simulink model "sim_test2"  (R2018a)
settings: Solver=FixedStepDiscrete  StartTime=0.0  StopTime=2e-3  FixedStep=Ts  RelTol=1e-3
InitFcn:
  | clear all;
  | close all;
  | clc;
  | 
  | Ts = 0.01e-3;  % sample period = 0.1 ms
  | Fs = 1/Ts;     % sample rate = 10kHz
settings Model: Creator=Ryan  LastModifiedBy=Ryan

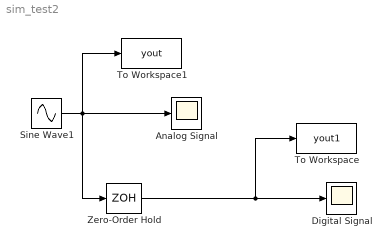
== system sim_test2 ==
  "Analog Signal " : Scope
  "Digital Signal " : Scope
  Sine Wave1 : Sin  Frequency=2*pi*1e3  SampleTime=0
  To Workspace : ToWorkspace  VariableName=yout1  SaveFormat=Structure With Time  SampleTime=-1
  To Workspace1 : ToWorkspace  VariableName=yout  SaveFormat=Structure With Time  SampleTime=-1
  Zero-Order Hold : ZeroOrderHold  SampleTime=10*Ts
  wires:
  Sine Wave1/1 -> To Workspace1/1, Zero-Order Hold/1, "Analog Signal "/1
  Zero-Order Hold/1 -> "Digital Signal "/1, To Workspace/1
